simulink model "w_to_attitude"  (R2019b)
settings: Solver=VariableStepAuto  StartTime=0.0  StopTime=10.0  RelTol=1e-3
settings Model: Creator=Tim  LastModifiedBy=Tim

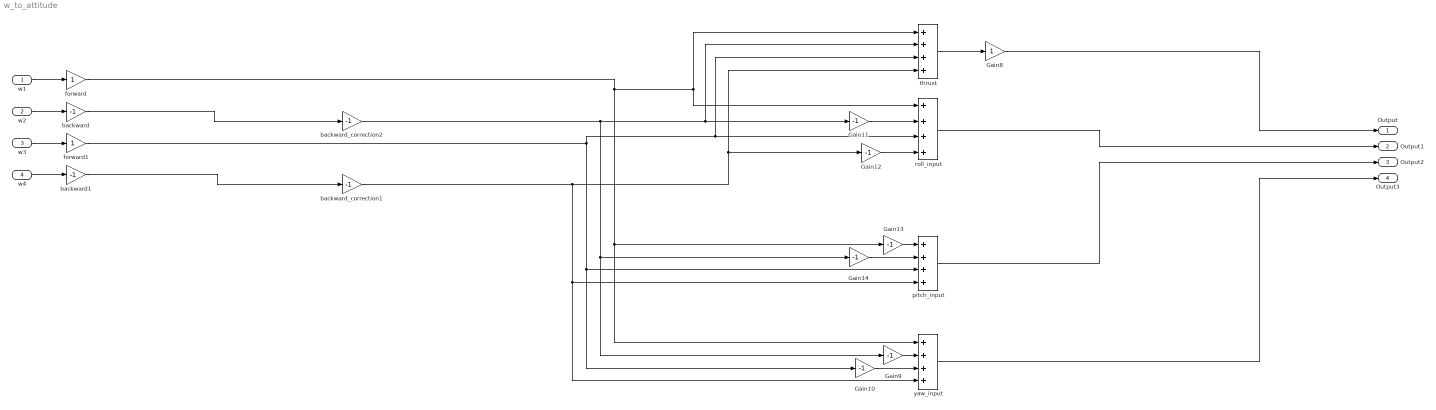
== system w_to_attitude ==
  w1 : Inport
  w2 : Inport  Port=2
  w3 : Inport  Port=3
  w4 : Inport  Port=4
  Gain{9..14} (6 alike) : Gain  Gain=-1
  Gain8 : Gain
  backward : Gain  Gain=-1
  backward1 : Gain  Gain=-1
  backward_correction1 : Gain  Gain=-1
  backward_correction2 : Gain  Gain=-1
  forward : Gain
  forward1 : Gain
  pitch_input : Sum  Inputs=++++
  roll_input : Sum  Inputs=++++
  thrust : Sum  Inputs=++++
  yaw_input : Sum  Inputs=++++
  Output : Outport
  Output1 : Outport  Port=2
  Output2 : Outport  Port=3
  Output3 : Outport  Port=4
  wires:
  backward_correction2/1 -> Gain9/1, Gain14/1, Gain11/1, thrust/2
  backward/1 -> backward_correction2/1
  Gain14/1 -> pitch_input/2
  Gain9/1 -> yaw_input/2
  Gain8/1 -> Output/1
  yaw_input/1 -> Output3/1
  Gain10/1 -> yaw_input/3
  Gain12/1 -> roll_input/4
  thrust/1 -> Gain8/1
  backward_correction1/1 -> thrust/4, Gain12/1, yaw_input/4, pitch_input/4
  w3/1 -> forward1/1
  w1/1 -> forward/1
  pitch_input/1 -> Output2/1
  Gain11/1 -> roll_input/2
  Gain13/1 -> pitch_input/1
  w2/1 -> backward/1
  forward1/1 -> Gain10/1, pitch_input/3, roll_input/3, thrust/3
  forward/1 -> Gain13/1, yaw_input/1, roll_input/1, thrust/1
  w4/1 -> backward1/1
  roll_input/1 -> Output1/1
  backward1/1 -> backward_correction1/1
